simulink model "PID_controller"  (R2023b)
settings: Solver=VariableStepAuto  StartTime=0.0  StopTime=10.0  RelTol=1e-3
libraries: cstblocks x3
settings Model: Creator=tinas  LastModifiedBy=tinas

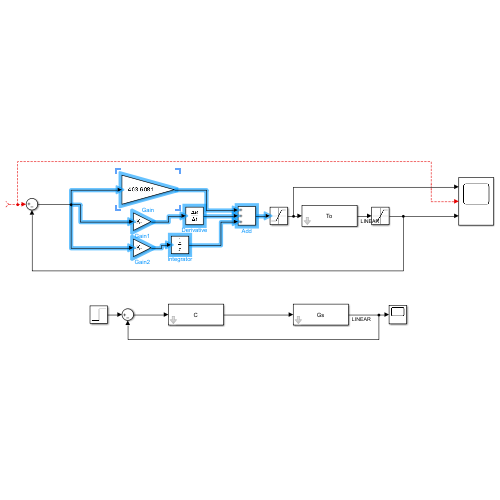
[thumbnail: Simulink's stored preview of the top-level diagram]
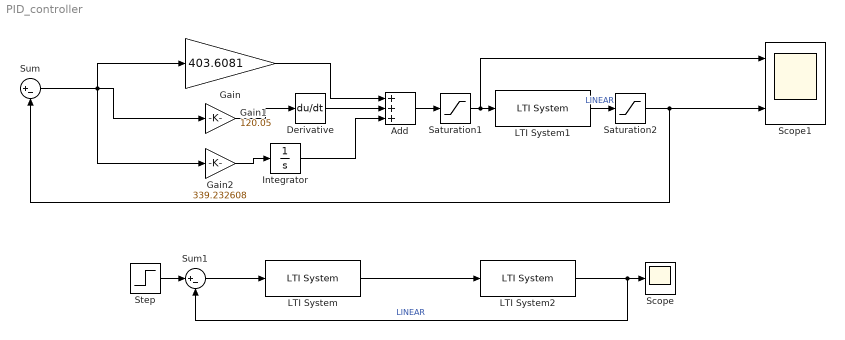
== system PID_controller ==
  Add : Sum  Inputs=+++
  Derivative : Derivative
  Gain : Gain  Gain=403.6081
  Gain1 : Gain  Gain=120.05
  Gain2 : Gain  Gain=339.232608
  Integrator : Integrator
  LTI System : cstblocks/LTI System  sys=C  IC=[]  PadeOrder=0
  LTI System1 : cstblocks/LTI System  sys=To  IC=[]  PadeOrder=0
  LTI System2 : cstblocks/LTI System  sys=Gs  IC=[]  PadeOrder=0
  Saturation1 : Saturate  UpperLimit=25  LowerLimit=-25
  Saturation2 : Saturate  UpperLimit=pi/2  LowerLimit=-pi/2
  Scope : Scope
  Scope1 : Scope  NumInputPorts=3
  Step : Step  SampleTime=0
  Sum : Sum  Inputs=|+-
  Sum1 : Sum  Inputs=|+-
  wires:
  ? -> Scope1/2, Sum/1
  Add/1 -> Saturation1/1
  Saturation1/1 -> Scope1/1, LTI System1/1
  Integrator/1 -> Add/3
  Saturation2/1 -> Sum/2, Scope1/3
  LTI System1/1 -> Saturation2/1  "LINEAR"
  Gain/1 -> Add/1
  Gain2/1 -> Integrator/1
  Gain1/1 -> Derivative/1
  Derivative/1 -> Add/2
  Sum/1 -> Gain2/1, Gain/1, Gain1/1
  LTI System/1 -> LTI System2/1
  LTI System2/1 -> Sum1/2, Scope/1  "LINEAR"
  Step/1 -> Sum1/1
  Sum1/1 -> LTI System/1
